simulink subsystem "s0606_SIL_observer"  (R2019b)
settings: Solver=VariableStepAuto  StartTime=0.0  StopTime=10.0  RelTol=1e-3
model mask{th_0=0, al_0=0, th_dot_0=0, al_dot_0=0}
  mask prompts: th_0 "Initial theta"; al_0 "Initial alpha"; th_dot_0 "Initial theta dot"; al_dot_0 "Initial alpha dot"
undefined symbols (not defined in the file): k_alpha, k_theta, PARAMS
settings Model: Creator=paolo  LastModifiedBy=giaco
settings DebuggingCC: SFMachineParentedDataDiag=error

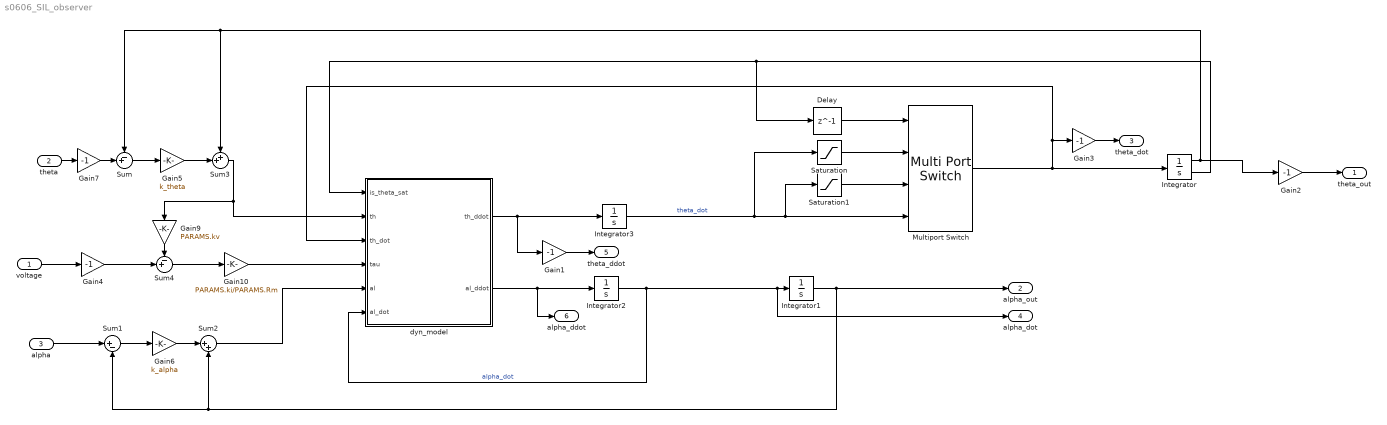
== system s0606_SIL_observer ==
  voltage : Inport  Unit=N*m  PortDimensions=1
  theta : Inport  Port=2  Unit=N*m  PortDimensions=1
  alpha : Inport  Port=3  Unit=N*m  PortDimensions=1
  Delay : Delay  DelayLength=1
  Gain{1..4,7} (5 alike) : Gain  Gain=-1
  Gain10 : Gain  Gain=PARAMS.ki/PARAMS.Rm
  Gain5 : Gain  Gain=k_theta
  Gain6 : Gain  Gain=k_alpha
  Gain9 : Gain  Gain=PARAMS.kv
  Integrator : Integrator  InitialCondition=th_0  LimitOutput=on  UpperSaturationLimit=135/180*pi  LowerSaturationLimit=-135/180*pi  ShowSaturationPort=on
  Integrator1 : Integrator  InitialCondition=al_0  UpperSaturationLimit=0.01  LowerSaturationLimit=-0.01
  Integrator2 : Integrator  InitialCondition=al_dot_0  UpperSaturationLimit=0.01  LowerSaturationLimit=-0.01
  Integrator3 : Integrator  InitialCondition=th_dot_0  UpperSaturationLimit=0.001  LowerSaturationLimit=-0.001
  Multiport Switch : MultiPortSwitch  DataPortOrder=Specify indices  DataPortIndices={-1,1,0}
  Saturation : Saturate  UpperLimit=inf  LowerLimit=0
  Saturation1 : Saturate  UpperLimit=0  LowerLimit=-inf
  Sum : Sum  Inputs=-+|
  Sum1 : Sum  Inputs=|+-
  Sum2 : Sum  Inputs=|++
  Sum3 : Sum  Inputs=++|
  Sum4 : Sum  Inputs=-+|
  dyn_model : MATLAB Function  TreatAsAtomicUnit=on
  "theta_out " : Outport  Unit=rad  PortDimensions=1
  alpha_out : Outport  Port=2  Unit=rad  PortDimensions=1
  theta_dot : Outport  Port=3  Unit=rad/s  PortDimensions=1
  alpha_dot : Outport  Port=4  Unit=rad/s  PortDimensions=1
  theta_ddot : Outport  Port=5  Unit=rad/s  PortDimensions=1
  alpha_ddot : Outport  Port=6  Unit=rad/s  PortDimensions=1
  wires:
  Integrator2/1 -> dyn_model/6(al_dot), Integrator1/1, alpha_dot/1  "alpha_dot"
  Integrator3/1 -> Multiport Switch/4, Saturation1/1, Saturation/1  "theta_dot"
  dyn_model/1(th_ddot) -> Gain1/1, Integrator3/1
  dyn_model/2(al_ddot) -> Integrator2/1, alpha_ddot/1
  voltage/1 -> Gain4/1
  Gain2/1 -> "theta_out "/1
  Integrator/2 -> dyn_model/1(is_theta_sat), Delay/1
  Multiport Switch/1 -> Gain3/1, dyn_model/3(th_dot), Integrator/1
  Delay/1 -> Multiport Switch/1
  Saturation/1 -> Multiport Switch/2
  Saturation1/1 -> Multiport Switch/3
  Integrator1/1 -> Sum2/2, Sum1/2, alpha_out/1
  Gain3/1 -> theta_dot/1
  Integrator/1 -> Sum/1, Sum3/1, Gain2/1
  theta/1 -> Gain7/1
  Sum/1 -> Gain5/1
  Gain5/1 -> Sum3/2
  Sum3/1 -> dyn_model/2(th), Gain9/1
  alpha/1 -> Sum1/1
  Sum1/1 -> Gain6/1
  Gain6/1 -> Sum2/1
  Sum2/1 -> dyn_model/5(al)
  Gain7/1 -> Sum/2
  Gain4/1 -> Sum4/2
  Gain9/1 -> Sum4/1
  Sum4/1 -> Gain10/1
  Gain10/1 -> dyn_model/4(tau)
  Gain1/1 -> theta_ddot/1

== matlab function s0606_SIL_observer/dyn_model ==
  data: is_theta_sat input; th input; th_dot input size=1; tau input size=1; th_ddot output; al input size=1; al_dot input size=1; al_ddot output size=1; PARAMS parameter
function [th_ddot, al_ddot] = dyn_model(is_theta_sat, th, th_dot, tau, al, al_dot, PARAMS)
    
    l1 = PARAMS.l1;
    l2 = PARAMS.l2;
    mp = PARAMS.mp;
    Lp = PARAMS.Lp;
    mr = PARAMS.mr;
    Lr = PARAMS.Lr;
    Jm = PARAMS.Jm;
    Jh = PARAMS.Jh;
    Cth = PARAMS.Cth;
    Cal = PARAMS.Cal;
    Dth = PARAMS.Dth;
    K = PARAMS.K;
    Sth = PARAMS.Sth;
    th_0 = PARAMS.th_0_cable;
    
    if is_theta_sat == 1 % theta clamped at 135 deg
        if tau > K*(th-th_0)
            tau = K*(th-th_0);
        end
    elseif is_theta_sat == -1 % theta clamped at -135 deg
        if tau < K*(th-th_0)
            tau = K*(th-th_0);
        end
    end

    if abs(th_dot) < PARAMS.Sth_vel_threshold
        if abs(tau - K*(th-th_0)) < Sth
            tau_static_friction = tau - K*(th-th_0);
        else
            tau_static_friction = Sth;
        end
        tau_dynamic_friction = 0;
    else
        tau_static_friction = 0;
        tau_dynamic_friction = Dth*sign(th_dot);
    end
    
    tau_actual = tau - tau_static_friction - tau_dynamic_friction;
    g = 9.81;
    
   th_ddot = (12*Lp^2*tau_actual + 144*l2^2*tau_actual - 12*Cth*Lp^2*th_dot - 12*K*Lp^2*th - 144*Cth*l2^2*th_dot - 144*K*l2^2*th + 144*Lr*al_dot^2*l2^3*mp*sin(al) + 72*Lr*g*l2^2*mp*sin(2*al) + 144*Cal*Lr*al_dot*l2*cos(al) - Lp^4*al_dot*mp*th_dot*sin(2*al) - 144*al_dot*l2^4*mp*th_dot*sin(2*al) + 144*Lr*l2^3*mp*th_dot^2*sin(al)*(sin(al)^2 - 1) - 24*Lp^2*al_dot*l2^2*mp*th_dot*sin(2*al) + 12*Lp^2*Lr*al_dot^2*l2*mp*sin(al) + 12*Lp^2*Lr*l2*mp*th_dot^2*sin(al)*(sin(al)^2 - 1))/(12*Jh*Lp^2 + 12*Jm*Lp^2 + 144*Jh*l2^2 + 144*Jm*l2^2 + 12*Lp^2*Lr^2*mp + Lp^2*Lr^2*mr + 12*Lp^2*l1^2*mr + 12*Lr^2*l2^2*mr + 144*l1^2*l2^2*mr + Lp^4*mp*sin(al)^2 + 144*l2^4*mp*sin(al)^2 + 24*Lp^2*l2^2*mp*sin(al)^2 + 144*Lr^2*l2^2*mp*sin(al)^2);
   al_ddot = -(144*Cal*Jh*al_dot + 144*Cal*Jm*al_dot + 144*Cal*Lr^2*al_dot*mp + 12*Cal*Lr^2*al_dot*mr + 144*Cal*al_dot*l1^2*mr + 144*g*l2^3*mp^2*sin(al)^3 + 12*Cal*Lp^2*al_dot*mp*sin(al)^2 + 144*Cal*al_dot*l2^2*mp*sin(al)^2 + 144*Lr^2*g*l2*mp^2*sin(al) - 6*Lp^2*Lr^2*mp^2*th_dot^2*sin(2*al) + 72*Lr^2*al_dot^2*l2^2*mp^2*sin(2*al) - Lp^4*mp^2*th_dot^2*cos(al)*sin(al)^3 - 72*Lr^2*l2^2*mp^2*th_dot^2*sin(2*al) + 144*Lr*l2*mp*tau_actual*cos(al) + 144*Jh*g*l2*mp*sin(al) + 144*Jm*g*l2*mp*sin(al) - 144*l2^4*mp^2*th_dot^2*cos(al)*sin(al)^3 - 6*Jh*Lp^2*mp*th_dot^2*sin(2*al) - 6*Jm*Lp^2*mp*th_dot^2*sin(2*al) + 12*Lp^2*g*l2*mp^2*sin(al)^3 - 72*Jh*l2^2*mp*th_dot^2*sin(2*al) - 72*Jm*l2^2*mp*th_dot^2*sin(2*al) - 144*Cth*Lr*l2*mp*th_dot*cos(al) - 144*K*Lr*l2*mp*th*cos(al) - 24*Lp^2*l2^2*mp^2*th_dot^2*cos(al)*sin(al)^3 + 12*Lr^2*g*l2*mp*mr*sin(al) - (Lp^2*Lr^2*mp*mr*th_dot^2*sin(2*al))/2 + 144*g*l1^2*l2*mp*mr*sin(al) - 6*Lp^2*l1^2*mp*mr*th_dot^2*sin(2*al) - 6*Lr^2*l2^2*mp*mr*th_dot^2*sin(2*al) - 72*l1^2*l2^2*mp*mr*th_dot^2*sin(2*al) + 288*Lr*al_dot*l2^3*mp^2*th_dot*sin(al)*(sin(al)^2 - 1) + 24*Lp^2*Lr*al_dot*l2*mp^2*th_dot*sin(al)*(sin(al)^2 - 1))/(mp*(12*Jh*Lp^2 + 12*Jm*Lp^2 + 144*Jh*l2^2 + 144*Jm*l2^2 + 12*Lp^2*Lr^2*mp + Lp^2*Lr^2*mr + 12*Lp^2*l1^2*mr + 12*Lr^2*l2^2*mr + 144*l1^2*l2^2*mr + Lp^4*mp*sin(al)^2 + 144*l2^4*mp*sin(al)^2 + 24*Lp^2*l2^2*mp*sin(al)^2 + 144*Lr^2*l2^2*mp*sin(al)^2));
 
    
end
